simulink model "furuta_model"  (R2020a)
settings: Solver=VariableStepAuto  StartTime=0.0  StopTime=10.0  RelTol=1e-3
PostLoadFcn:
  | m_p = 0.3;  %pendulum mass [kg]
  | l_p = 0.205;  %pendulum length [m]
  | m_b = 1;  %brace mass [kg]
  | l_b = 0.3;  %brace length [m]
  | M = 1;  %puntiform mass [kg]
  | J = 0.1531;  %moment of inertia [kg*m^2]
  | g = 9.81;  %gravity [m*s^-2]
  | 
  | k = 2.7;  %torque drive constant [Nm/V]
  | k_i = 2.667;  %drive transconductance constant [A/V]
  | k_g = 15;  %trasmission ratio
  | k_t = 0.1;  %torque motor constant [Nm/A]
  | 
  | b_phi = 0.337;  %viscous friction of brace [Nm s/rad]
  | b_theta = 0.035;  %viscous friction of pendulum [Nm s/rad]
settings Model: Creator=angelo  LastModifiedBy=angelo

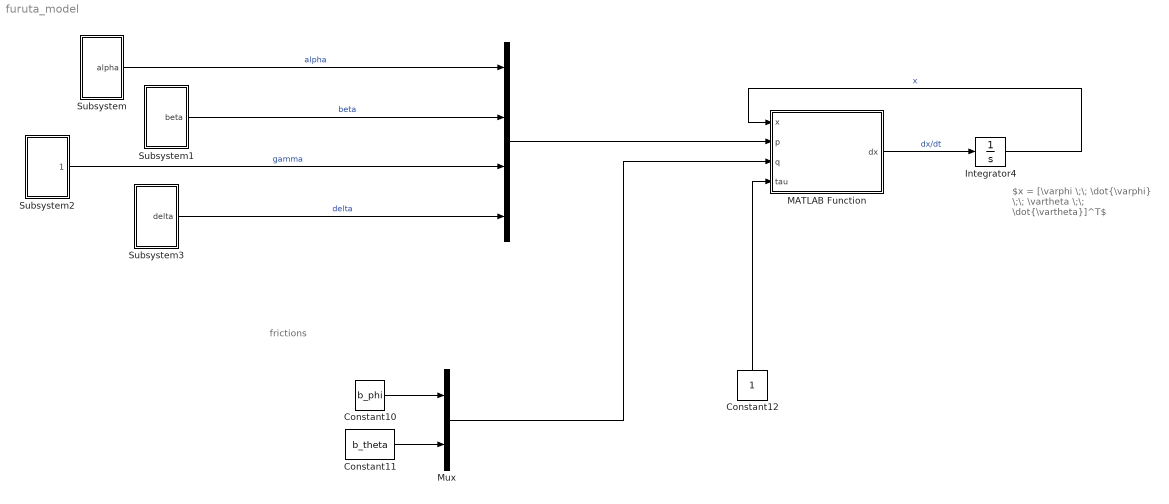
== system furuta_model ==
  note: frictions
  note: $x = [\varphi \;\; \dot{\varphi} \;\; \vartheta \;\; \dot{\vartheta}]^T$
  " " : Mux
  Constant10 : Constant  Value=b_phi
  Constant11 : Constant  Value=b_theta
  Constant12 : Constant
  Integrator4 : Integrator
  MATLAB Function : MATLAB Function  TreatAsAtomicUnit=on
  Mux : Mux  Inputs=2
  Subsystem : Subsystem
  Subsystem1 : Subsystem
  Subsystem2 : Subsystem
  Subsystem3 : Subsystem
  wires:
  " "/1 -> MATLAB Function/2(p)
  Constant10/1 -> Mux/1
  Constant11/1 -> Mux/2
  Mux/1 -> MATLAB Function/3(q)
  Constant12/1 -> MATLAB Function/4(tau)
  MATLAB Function/1(dx) -> Integrator4/1  "dx/dt"
  Integrator4/1 -> MATLAB Function/1(x)  "x"
  Subsystem/1(alpha) -> " "/1  "alpha"
  Subsystem1/1(beta) -> " "/2  "beta"
  Subsystem2/1(gamma) -> " "/3  "gamma"
  Subsystem3/1(delta) -> " "/4  "delta"

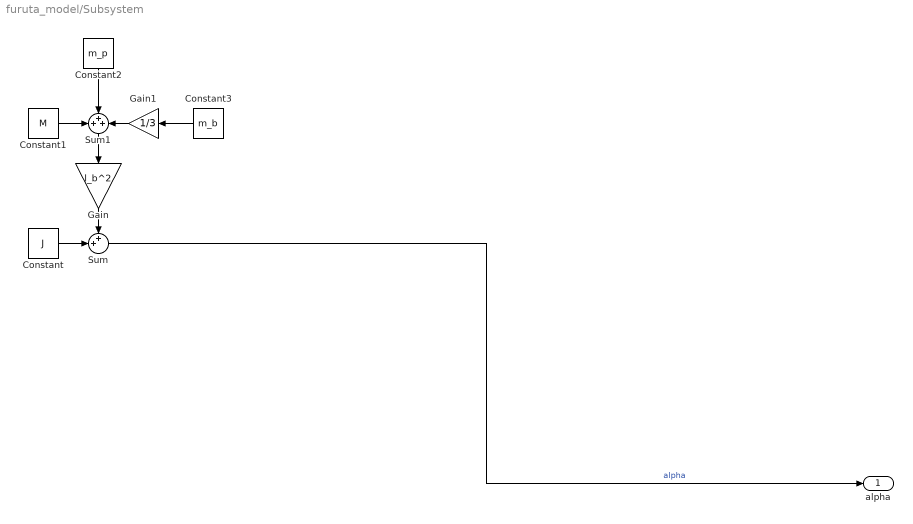
== system furuta_model/Subsystem ==
  Constant : Constant  Value=J
  Constant1 : Constant  Value=M
  Constant2 : Constant  Value=m_p
  Constant3 : Constant  Value=m_b
  Gain : Gain  Gain=l_b^2
  Gain1 : Gain  Gain=1/3
  Sum : Sum  Inputs=++|
  Sum1 : Sum  Inputs=+++
  alpha : Outport
  wires:
  Constant1/1 -> Sum1/1
  Constant2/1 -> Sum1/2
  Gain1/1 -> Sum1/3
  Sum1/1 -> Gain/1
  Sum/1 -> alpha/1  "alpha"
  Constant/1 -> Sum/2
  Constant3/1 -> Gain1/1
  Gain/1 -> Sum/1

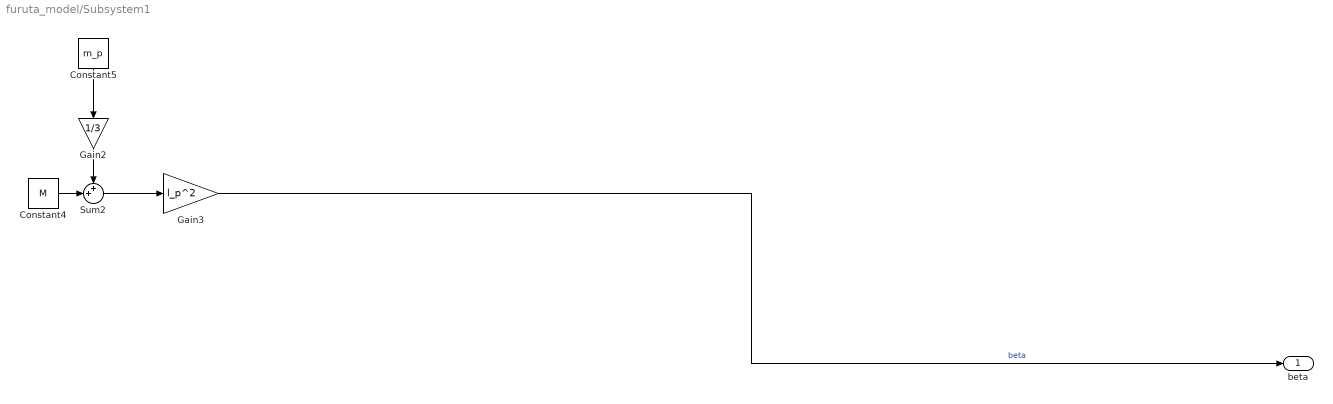
== system furuta_model/Subsystem1 ==
  Constant4 : Constant  Value=M
  Constant5 : Constant  Value=m_p
  Gain2 : Gain  Gain=1/3
  Gain3 : Gain  Gain=l_p^2
  Sum2 : Sum  Inputs=++|
  beta : Outport
  wires:
  Constant5/1 -> Gain2/1
  Gain3/1 -> beta/1  "beta"
  Sum2/1 -> Gain3/1
  Constant4/1 -> Sum2/2
  Gain2/1 -> Sum2/1

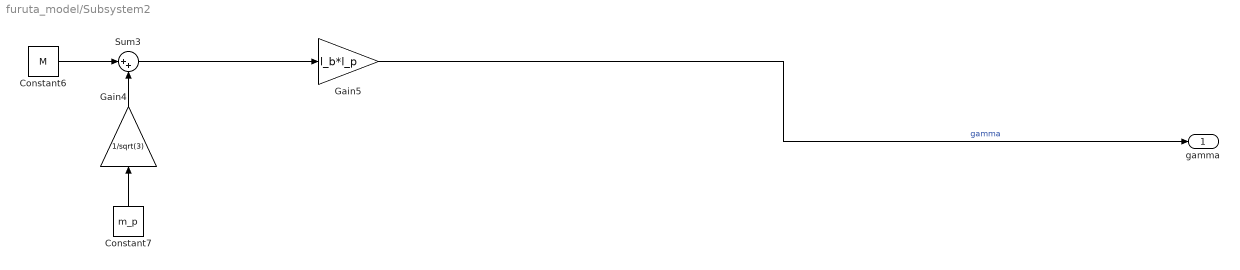
== system furuta_model/Subsystem2 ==
  Constant6 : Constant  Value=M
  Constant7 : Constant  Value=m_p
  Gain4 : Gain  Gain=1/sqrt(3)
  Gain5 : Gain  Gain=l_b*l_p
  Sum3 : Sum  Inputs=|++
  gamma : Outport
  wires:
  Constant6/1 -> Sum3/1
  Gain5/1 -> gamma/1  "gamma"
  Sum3/1 -> Gain5/1
  Gain4/1 -> Sum3/2
  Constant7/1 -> Gain4/1

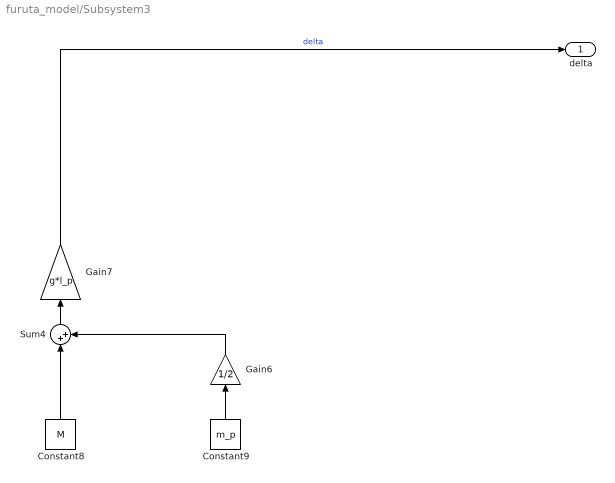
== system furuta_model/Subsystem3 ==
  Constant8 : Constant  Value=M
  Constant9 : Constant  Value=m_p
  Gain6 : Gain  Gain=1/2
  Gain7 : Gain  Gain=g*l_p
  Sum4 : Sum  Inputs=|++
  delta : Outport
  wires:
  Gain6/1 -> Sum4/2
  Gain7/1 -> delta/1  "delta"
  Sum4/1 -> Gain7/1
  Constant8/1 -> Sum4/1
  Constant9/1 -> Gain6/1

== matlab function furuta_model/MATLAB Function ==
  data: x input; dx output; p input; q input; tau input
function dx = furuta(x, p, q, tau)
% p = parameters vector
% q = frictions vector
% si sconsiglia di avere variabili globali nelle function

x = zeros(4, 1);

% parameters
alpha = p(1);
beta = p(2);
gamma = p(3);
delta = p(4);

% frictions
b_phi = q(1);
b_theta = q(2);

% state
phi = x(1);
dphi = x(2);
theta = x(3);  
dtheta = x(4);

% input
tau_phi = tau;
%tau_phi = tau(1);
%tau_theta = tau(2);

% common term for ddphi and ddtheta
t0 = 1/(beta*(alpha + beta*sin(theta)^2)-gamma^2*cos(theta)^2);

% terms of ddphi
t1 = beta*gamma*sin(theta)*dtheta^2;
t2 = gamma*delta*cos(theta)*sin(theta);
t3 = (2*beta^2*cos(theta)*sin(theta))*dphi*dtheta;
t4 = gamma*b_theta*cos(theta)*dtheta;
t5 = (beta*gamma*cos(theta)^2*sin(theta))*dphi^2;
t6 = beta*(tau_phi - b_phi*dphi);

% ddphi
ddphi = t0*(t1-t2-t3+t4+t5+t6);

% terms of ddtheta
t00 = (alpha + beta*sin(theta)^2);
t1 = t00*delta*sin(theta);
t2 = t00*(beta*cos(theta)*sin(theta)*dphi^2);
t3 = 2*beta*gamma*cos(theta)^2*sin(theta)*dphi*dtheta;
t4 = gamma^2*sin(theta)*cos(theta)*dtheta^2;
t5 = t00*b_theta*dtheta;
t6 = gamma*cos(theta)*b_theta*dphi;
t7 = gamma*cos(theta)*tau_phi;

% ddtheta
ddtheta = t0*(t1 +t2 +t3 - t4 - t5 + t6 - t7);

% output
dx = zeros(4, 1);
dx(1) = dphi;
dx(2) = ddphi;
dx(3) = dtheta;
dx(4) = ddtheta;
